simulink model "Eg3_3"  (R2018a)
settings: Solver=VariableStepAuto  StartTime=0.0  StopTime=10.0  RelTol=1e-3
libraries: simulink x1
settings Model: Creator=wangluo  LastModifiedBy=wangluo

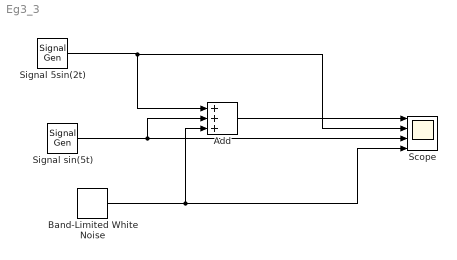
== system Eg3_3 ==
  Add : Sum  Inputs=+++
  Band-Limited White Noise : simulink/Sources/Band-Limited White Noise  Cov=[0.5]  Ts=0.1  seed=[23341]
  Scope : Scope  NumInputPorts=4
  Signal 5sin(2t) : SignalGenerator  Amplitude=5  Frequency=2  Units=rad/sec
  Signal sin(5t) : SignalGenerator  Frequency=5  Units=rad/sec
  wires:
  Signal 5sin(2t)/1 -> Scope/2, Add/1
  Signal sin(5t)/1 -> Add/2, Scope/3
  Add/1 -> Scope/1
  Band-Limited White Noise/1 -> Scope/4, Add/3
